simulink model "Holder"  (R2013a)
settings: Solver=ode45  StartTime=0.0  StopTime=10.0  RelTol=1e-3
undefined symbols (not defined in the file): timeconst, Ts
settings Model: Creator=Sam  LastModifiedBy=Sam

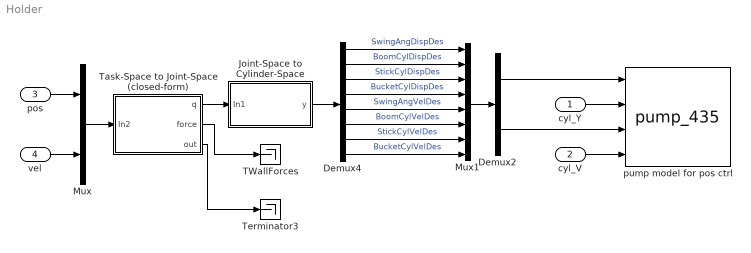
== system Holder ==
  cyl_Y : Inport
  cyl_V : Inport  Port=2
  pos : Inport  Port=3
  vel : Inport  Port=4
  Demux2 : Demux  Outputs=2
  Demux4 : Demux  Outputs=8
  Joint-Space to Cylinder-Space : Subsystem  mask{SI=on, Ts=Ts}
      mask prompts: SI "Use SI units"; Ts "Sampling Time"
      mask Display:
      | port_label('input',1,'J')
      | port_label('output',1,'C')
      | fprintf('J2C')
  Mux : Mux  Inputs=2
  Mux1 : Mux  Inputs=8
  TWallForces : Terminator
  Task-Space to Joint-Space (closed-form) : Subsystem  mask{SI=on, distal_flag=off, Ts=Ts}
      mask prompts: SI "Use SI units"; distal_flag "Distal Bucket Control"; Ts "Sampling Time"
      mask Display:
      | port_label('input',1,'T')
      | port_label('output',1,'J')
      | port_label('output',2,'Force')
      | fprintf('T2J')
  Terminator3 : Terminator
  pump model for pos ctrl : S-Function  FunctionName=pump_435  Parameters=Ts, tau, pgain1, pgain2, pgain3, pgain4, vgain1, vgain2, vgain3, vgain4  EnableBusSupport=off  mask{Ts=Ts, tau=timeconst, pgain1=-80, pgain2=-20, pgain3=-20, pgain4=-20, vgain1=-30, vgain2=-.1, vgain3=-.1, vgain4=-.1}
      mask prompts: Ts "Sampling time"; tau "Time constant"; pgain1 "Swing position gain"; pgain2 "Boom position gain"; pgain3 "Arm position gain"; pgain4 "Bucket position gain"; vgain1 "Swing velocity gain"; vgain2 "Boom velocity gain"; vgain3 "Arm velocity gain"; vgain4 "Bucket velocity gain"
      mask Display:
      | port_label('input',1,'ydes')
      | port_label('input',2,'y')
      | port_label('input',3,'vdes')
      | port_label('input',4,'v')
      | 
      | port_label('output',1,'Flow')
      | 
      | fprintf('Pump')
  wires:
  Demux2/1 -> pump model for pos ctrl/1
  cyl_V/1 -> pump model for pos ctrl/4
  cyl_Y/1 -> pump model for pos ctrl/2
  vel/1 -> Mux/2
  Demux4/3 -> Mux1/3  "StickCylDispDes"
  Demux4/4 -> Mux1/4  "BucketCylDispDes"
  Demux4/5 -> Mux1/5  "SwingAngVelDes"
  Demux4/6 -> Mux1/6  "BoomCylVelDes"
  Demux4/7 -> Mux1/7  "StickCylVelDes"
  Demux4/8 -> Mux1/8  "BucketCylVelDes"
  Demux4/1 -> Mux1/1  "SwingAngDispDes"
  Demux4/2 -> Mux1/2  "BoomCylDispDes"
  Joint-Space to Cylinder-Space/1(y) -> Demux4/1
  Mux1/1 -> Demux2/1
  Task-Space to Joint-Space (closed-form)/1(q) -> Joint-Space to Cylinder-Space/1(In1)
  Task-Space to Joint-Space (closed-form)/2(force) -> TWallForces/1
  Mux/1 -> Task-Space to Joint-Space (closed-form)/1(In2)
  Task-Space to Joint-Space (closed-form)/3(out) -> Terminator3/1
  pos/1 -> Mux/1
  Demux2/2 -> pump model for pos ctrl/3

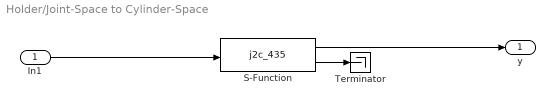
== system Holder/Joint-Space to Cylinder-Space ==
  In1 : Inport
  S-Function : S-Function  FunctionName=j2c_435  Parameters=Ts  EnableBusSupport=off
  Terminator : Terminator
  y : Outport
  wires:
  S-Function/1 -> y/1
  In1/1 -> S-Function/1
  S-Function/2 -> Terminator/1

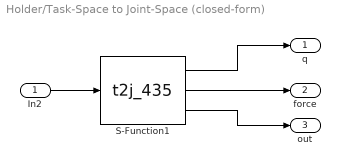
== system Holder/Task-Space to Joint-Space (closed-form) ==
  In2 : Inport
  S-Function1 : S-Function  FunctionName=t2j_435  Parameters=Ts  EnableBusSupport=off
  q : Outport
  force : Outport  Port=2
  out : Outport  Port=3
  wires:
  S-Function1/1 -> q/1
  In2/1 -> S-Function1/1
  S-Function1/2 -> force/1
  S-Function1/3 -> out/1
